simulink model "UZ_EnDat_be4_optimizing_ctrs"  (R2023b)
settings: Solver=FixedStepDiscrete  StartTime=0  StopTime=0.002  RelTol=1e-3
model workspace (MAT data in the model file):
  Select = 0
libraries: hdlsllib x755, simulink x20, simulink_extras x4
(part 1 of 9)
settings Model: DataTypeOverride=Off  SimulationMode=accelerator  NumberOfSteps=10  PacingRate=1000  Creator=ELSYS_PC  LastModifiedBy=ELSYS_PC
settings SolverCC: AlgebraicLoopSolver=TrustRegion
settings DataIOCC: LimitDataPoints=on  SaveOutput=off  SaveTime=off
settings OptimizationCC: BlockReduction=off  ConditionallyExecuteInputs=off  DefaultParameterBehavior=Inlined  InheritOutputTypeSmallerThanSingle=on  LifeSpan=inf
settings DebuggingCC: AlgebraicLoopMsg=error  SingleTaskRateTransMsg=error  UnconnectedInputMsg=warning  UnconnectedOutputMsg=warning  UnconnectedLineMsg=warning  AllowSymbolicDim=off  StrictBusMsg=ErrorOnBusTreatedAsVector  SFUnexpectedBacktrackingDiag=warning  SFNoUnconditionalDefaultTransitionDiag=warning  SFExecutionAtInitializationDiag=none  ArithmeticOperatorsInVariantConditions=warning
settings HardwareCC: ProdBitPerPointer=32  ProdBitPerSizeT=32  ProdBitPerPtrDiffT=32  ProdLargestAtomicFloat=None  ProdIntDivRoundTo=Undefined  ProdEndianess=Unspecified  ProdWordSize=32  ProdHWDeviceType=ASIC/FPGA->ASIC/FPGA  TargetBitPerPointer=64  TargetBitPerSizeT=64  TargetBitPerPtrDiffT=64  TargetLongLongMode=on  TargetIntDivRoundTo=Zero  TargetEndianess=LittleEndian  TargetWordSize=64  TargetHWDeviceType=Custom Processor->MATLAB Host Computer  ProdEqTarget=off
settings ModelReferenceCC: EnableRefExpFcnMdlSchedulingChecks=on
settings SFSimCC: SimUseLocalCustomCode=off  CustomCodeUndefinedFunction=UseInterfaceOnly
settings RTWCC: RTWUseLocalCustomCode=off
settings CodeAppCC: StateflowObjectComments=on
settings GRTTargetCC: TargetLangStandard=C89/C90 (ANSI)  RTWCAPISignals=on  RTWCAPIParams=on
settings ConfigComp: CovScope=ReferencedModels  CovMetricSettings=dw  CovSaveCumulativeToWorkspaceVar=on  CovSaveSingleToWorkspaceVar=on  CovExternalEMLEnable=off  CovSFcnEnable=off  DVTestSuiteOptimization=Auto  DVDetectOutOfBounds=on  DVModelReferenceHarness=on  DVHarnessSource=Signal Editor  DVRebuildModelRepresentation=IfChangeIsDetected

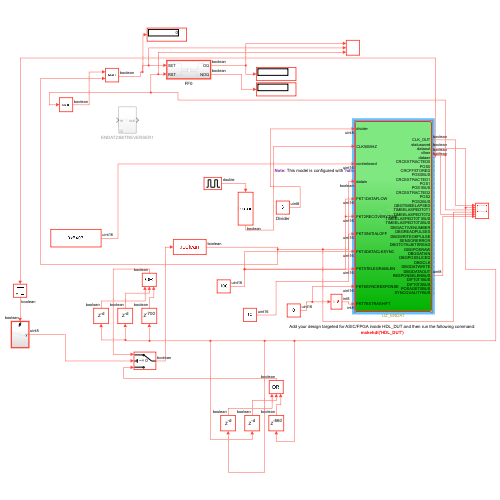
[thumbnail: Simulink's stored preview of the top-level diagram]
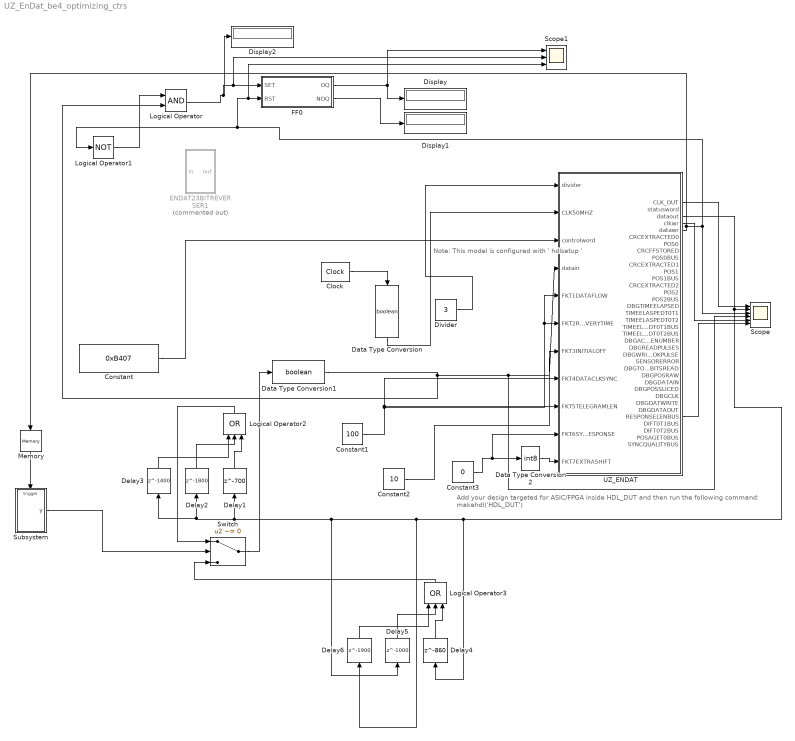
== system UZ_EnDat_be4_optimizing_ctrs ==
  note: Note: This model is configured with ' hdlsetup '
  note: Add your design targeted for ASIC/FPGA inside HDL_DUT and then run the following command:
      | makehdl('HDL_DUT')
  Clock : simulink_extras/Flip Flops/Clock  period=2E-8
  Constant : Constant  Value=0xB407  OutDataTypeStr=uint16  SampleTime=-1
  Constant1 : Constant  Value=100  OutDataTypeStr=uint16  SampleTime=-1
  Constant2 : Constant  Value=10  OutDataTypeStr=uint16  SampleTime=-1
  Constant3 : Constant  Value=0  OutDataTypeStr=uint16  SampleTime=-1
  Data Type Conversion : DataTypeConversion  OutDataTypeStr=boolean  SaturateOnIntegerOverflow=off  RndMeth=Floor
  Data Type Conversion1 : DataTypeConversion  OutDataTypeStr=boolean  SaturateOnIntegerOverflow=off  RndMeth=Floor
  Data Type Conversion2 : DataTypeConversion  OutDataTypeStr=int8  SaturateOnIntegerOverflow=off  RndMeth=Floor
  Delay1 : Delay  DelayLength=700
  Delay2 : Delay  DelayLength=1800
  Delay3 : Delay  DelayLength=1400
  Delay4 : Delay  DelayLength=860
  Delay5 : Delay  DelayLength=1000
  Delay6 : Delay  DelayLength=1900
  Display : Display
  Display1 : Display
  Display2 : Display
  Divider : Constant  Value=3  OutMin=0  OutMax=7  OutDataTypeStr=uint8  SampleTime=-1
  ENDAT23BITREVERSER1 : Subsystem  Commented=on
  FF0 : Subsystem  TreatAsAtomicUnit=on
      settings: LibrarySourceBlock=|
      | hdlsllib/Ports &
      | Subsystems/Triggered
      | Subsystem
  Logical Operator : Logic  AllPortsSameDT=off  OutDataTypeStr=boolean
  Logical Operator1 : Logic  Operator=NOT  AllPortsSameDT=off  OutDataTypeStr=boolean
  Logical Operator2 : Logic  Operator=OR  Inputs=3  AllPortsSameDT=off  OutDataTypeStr=boolean
  Logical Operator3 : Logic  Operator=OR  Inputs=3  AllPortsSameDT=off  OutDataTypeStr=boolean
  Memory : Memory  InheritSampleTime=on
  Scope : Scope  NumInputPorts=6
  Scope1 : Scope  NumInputPorts=3
  Subsystem : Subsystem
  Switch : Switch  Criteria=u2 ~= 0  SaturateOnIntegerOverflow=off  InputSameDT=off
  UZ_ENDAT : Subsystem  TreatAsAtomicUnit=on
  wires:
  Constant/1 -> UZ_ENDAT/3(controlword)
  Data Type Conversion/1 -> UZ_ENDAT/2(CLK50MHZ)
  Divider/1 -> UZ_ENDAT/1(divider)
  Clock/1 -> Data Type Conversion/1
  Data Type Conversion1/1 -> Logical Operator/2, Scope/4, UZ_ENDAT/4(datain)
  Delay1/1 -> Logical Operator2/3
  UZ_ENDAT/1(CLK_OUT) -> Scope/1
  UZ_ENDAT/5(datawr) -> Memory/1, Scope1/3, FF0/2(RST), Logical Operator1/1, Scope/3
  Constant1/1 -> UZ_ENDAT/5(FKT1DATAFLOW), UZ_ENDAT/6(FKT2RECOVERYTIME), UZ_ENDAT/8(FKT4DATACLKSYNC), UZ_ENDAT/9(FKT5TELEGRAMLEN)
  Constant2/1 -> UZ_ENDAT/7(FKT3INITIALOFF)
  FF0/1(OQ) -> Scope1/1, Display/1
  Logical Operator/1 -> Scope1/2, FF0/1(SET), Display2/1
  FF0/2(NOQ) -> Display1/1
  Logical Operator1/1 -> Logical Operator/1
  Delay2/1 -> Logical Operator2/2
  Delay3/1 -> Logical Operator2/1
  Logical Operator2/1 -> Switch/1
  Switch/1 -> Data Type Conversion1/1
  Delay6/1 -> Logical Operator3/1
  Delay5/1 -> Logical Operator3/2
  Logical Operator3/1 -> Switch/3
  Delay4/1 -> Logical Operator3/3
  UZ_ENDAT/3(dataout) -> Delay4/1, Delay6/1, Delay3/1, Delay2/1, Delay1/1, Delay5/1, Scope/2
  Subsystem/1(y) -> Switch/2
  Memory/1 -> Subsystem/Trigger
  UZ_ENDAT/4(clkwr) -> Scope/5
  Constant3/1 -> UZ_ENDAT/10(FKT6SYNCRESPONSE), Data Type Conversion2/1
  Data Type Conversion2/1 -> UZ_ENDAT/11(FKT7EXTRASHIFT)
  UZ_ENDAT/32(RESPONSELENBUS) -> Scope/6

== system UZ_EnDat_be4_optimizing_ctrs/ENDAT23BITREVERSER1 ==
  in : Inport
  16BITREVERSER : Subsystem
  16BITREVERSER1 : Subsystem
  Bit Concat : hdlsllib/Logic and Bit Operations/Bit Concat  numInputs=2
  Bit Shift : hdlsllib/Logic and Bit Operations/Bit Shift  mode=Shift Right Logical  N=8
  Bit Slice : hdlsllib/Logic and Bit Operations/Bit Slice  lidx=15  ridx=0
  Bit Slice1 : hdlsllib/Logic and Bit Operations/Bit Slice  lidx=22  ridx=16
  out : Outport
  wires:
  Bit Concat/1 -> Bit Shift/1
  Bit Shift/1 -> out/1
  in/1 -> Bit Slice1/1, Bit Slice/1
  Bit Slice/1 -> 16BITREVERSER/1(in)
  Bit Slice1/1 -> 16BITREVERSER1/1(in)
  16BITREVERSER/1(out) -> Bit Concat/1
  16BITREVERSER1/1(out) -> Bit Concat/2

== system UZ_EnDat_be4_optimizing_ctrs/FF0 ==
  SET : Inport
  RST : Inport  Port=2
  S-R Flip-Flop : simulink_extras/Flip Flops/S-R Flip-Flop  initial_condition=0
  OQ : Outport
  NOQ : Outport  Port=2
  wires:
  SET/1 -> S-R Flip-Flop/1
  RST/1 -> S-R Flip-Flop/2
  S-R Flip-Flop/1 -> OQ/1
  S-R Flip-Flop/2 -> NOQ/1

== system UZ_EnDat_be4_optimizing_ctrs/Subsystem ==
  Trigger : TriggerPort  VariantControl=(inherit)  PortDimensions=1
  Counter Limited : hdlsllib/Sources/Counter Limited  uplimit=1  tsamp=-1
  y : Outport
  wires:
  Counter Limited/1 -> y/1

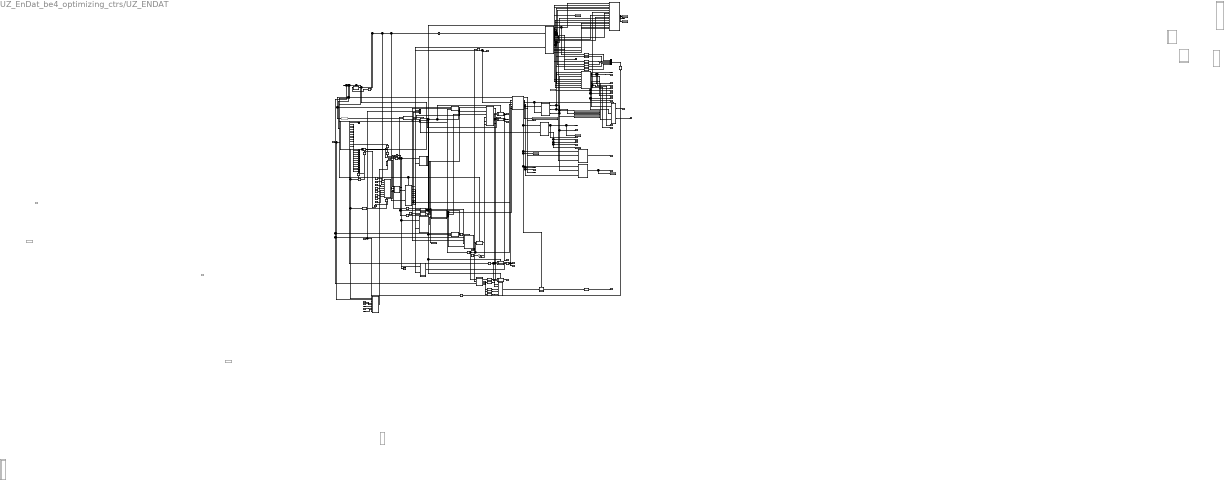
== system UZ_EnDat_be4_optimizing_ctrs/UZ_ENDAT ==
  note: 0=12.5;1=6,25;2=3,125;3=1,5625
  divider : Inport  OutDataTypeStr=uint8  SampleTime=1e-8
  CLK50MHZ : Inport  Port=2  SampleTime=1e-8
  controlword : Inport  Port=3  OutDataTypeStr=uint16  SampleTime=1e-8
  datain : Inport  Port=4  OutDataTypeStr=boolean  SampleTime=1e-8
  FKT1DATAFLOW : Inport  Port=5  OutDataTypeStr=uint16  SampleTime=1e-8
  FKT2RECOVERYTIME : Inport  Port=6  OutDataTypeStr=uint16  SampleTime=1e-8
  FKT3INITIALOFF : Inport  Port=7  OutDataTypeStr=uint16  SampleTime=1e-8
  FKT4DATACLKSYNC : Inport  Port=8  OutDataTypeStr=uint16  SampleTime=1e-8
  FKT5TELEGRAMLEN : Inport  Port=9  OutDataTypeStr=uint16  SampleTime=1e-8
  FKT6SYNCRESPONSE : Inport  Port=10  OutDataTypeStr=uint16  SampleTime=1e-8
  FKT7EXTRASHIFT : Inport  Port=11  OutDataTypeStr=int8  SampleTime=1e-8
  16BIT_SPLITTER1 : Subsystem  Commented=on  TreatAsAtomicUnit=on
  16bitgather : Subsystem
      settings: LibrarySourceBlock=|
      | hdlsllib/Ports &
      | Subsystems/Subsystem
  2CLKDELAY : Delay  DelayLengthSource=Input port  DelayLength=10  DelayLengthUpperLimit=127  PreventDirectFeedthrough=on
      settings: InputPortMap=u0,p1
  3timestorage : Subsystem
      settings: LibrarySourceBlock=|
      | hdlsllib/Ports &
      | Subsystems/Subsystem
  8BIT_SPLITTER : Subsystem  TreatAsAtomicUnit=on
  8BIT_SPLITTER1 : Subsystem  Commented=on  TreatAsAtomicUnit=on
  Bits to Word : hdlsllib/Logic and Bit Operations/Bits to Word
  CLKCNTER_ACT : Subsystem
      settings: LibrarySourceBlock=|
      | hdlsllib/Ports &
      | Subsystems/Subsystem
  CLKCNTER_NOSTOP : Subsystem
      settings: LibrarySourceBlock=|
      | hdlsllib/Ports &
      | Subsystems/Subsystem
  CLKDIV2 : Subsystem  Commented=through
  CLKGEN : Subsystem
  CONTROLWORDRAW : Subsystem
      settings: LibrarySourceBlock=|
      | hdlsllib/Ports &
      | Subsystems/Subsystem
  CONTROLWORDSTORED : Subsystem
      settings: LibrarySourceBlock=|
      | hdlsllib/Ports &
      | Subsystems/Subsystem
  CRC_Check : Subsystem  TreatAsAtomicUnit=on
  Compare To Constant : hdlsllib/Logic and Bit Operations/Compare To Constant  relop===  const=1  OutDataTypeStr=boolean
  Compare To Constant1 : hdlsllib/Logic and Bit Operations/Compare To Constant  relop===  const=1  OutDataTypeStr=boolean
  Compare To Constant2 : hdlsllib/Logic and Bit Operations/Compare To Constant  relop===  const=0  OutDataTypeStr=boolean
  Compare To Constant3 : hdlsllib/Logic and Bit Operations/Compare To Constant  relop=>=  const=3  OutDataTypeStr=boolean
  Constant10 : Constant  Commented=on  Value=3  OutDataTypeStr=fixdt(0,4,0)  SampleTime=-1
  Constant11 : Constant  Commented=on  Value=0xB407  OutDataTypeStr=uint16  SampleTime=-1
  Constant3 : Constant  OutDataTypeStr=boolean  SampleTime=-1
  Constant6 : Constant  Value=51  OutDataTypeStr=uint16  SampleTime=-1
  ControlWordRAM : Constant  Value=0  VectorParams1D=off  OutDataTypeStr=uint8  SampleTime=-1
  DATA2CLOCKSYNCER : Subsystem
  DATA2CLOCKSYNCER1 : Subsystem  Commented=on
  DATAFLOWCHGER : Subsystem
  DIFFBUILDER : Subsystem  TreatAsAtomicUnit=on
  Data Type Conversion : DataTypeConversion  OutDataTypeStr=fixdt(0,4,0)  RndMeth=Nearest
  Data Type Conversion1 : DataTypeConversion  OutDataTypeStr=uint8  SaturateOnIntegerOverflow=off  RndMeth=Floor
  Data Type Conversion{2..12} (11 alike) : DataTypeConversion  OutMax=1  OutDataTypeStr=fixdt(0,1)  SaturateOnIntegerOverflow=off  RndMeth=Floor
  Delay : Delay  DelayLength=10  InitialCondition=0
  Delay1 : Delay  DelayLengthSource=Input port  DelayLengthUpperLimit=127  InitialCondition=0
      settings: InputPortMap=u0,p1
  Delay2 : Delay  DelayLength=1
  Delay3 : Delay  DelayLength=1
  Detect Change : simulink/Logic and Bit Operations/Detect Change  vinit=0  OutDataTypeStr=boolean
      settings: LibrarySourceBlock=|
      | hdlsllib/Logic and Bit
      | Operations/Detect
      | Change
  Display{,1..6,8..11,14..15} (13 alike) : Display
      Display settings: Format=hex (Stored Integer)
      Display1 settings: Format=binary (Stored Integer)
      Display2 settings: Format=binary (Stored Integer)
      Display3 settings: Format=binary (Stored Integer)
      Display4 settings: Format=binary (Stored Integer)
      Display8 settings: Format=hex (Stored Integer)
      Display9 settings: Format=hex (Stored Integer)
  Dual Port RAM System : hdlsllib/HDL RAMs/Dual Port RAM System  RAMType=Dual port  AsyncRead=off  WriteOutputValue=New data  RAMInitialValue=0  allowBusInputs=off  WritesHaveOutput=on  NumReads=0  NumWrites=1  SimulateUsing=Code generation
  EndatControlRAM : Constant  VectorParams1D=off  OutDataTypeStr=uint8  SampleTime=-1
  FKT1 : Constant  Value=2  VectorParams1D=off  OutDataTypeStr=uint8  SampleTime=-1
  FKT2 : Constant  Value=3  VectorParams1D=off  OutDataTypeStr=uint8  SampleTime=-1
  FKT3 : Constant  Commented=on  Value=4  VectorParams1D=off  OutDataTypeStr=uint8  SampleTime=-1
  FKT4 : Constant  Value=5  VectorParams1D=off  OutDataTypeStr=uint8  SampleTime=-1
  FKT5 : Constant  Value=6  VectorParams1D=off  OutDataTypeStr=uint8  SampleTime=-1
  FKT6 : Constant  Value=7  VectorParams1D=off  OutDataTypeStr=uint8  SampleTime=-1
  FKT7 : Constant  Value=8  VectorParams1D=off  OutDataTypeStr=uint8  SampleTime=-1
  INITIALOFF : Subsystem
  Logical Operator : Logic  AllPortsSameDT=off  OutDataTypeStr=boolean
  Logical Operator1 : Logic  AllPortsSameDT=off  OutDataTypeStr=boolean
  Logical Operator10 : Logic  Operator=NOT  Inputs=3  AllPortsSameDT=off  OutDataTypeStr=boolean
  Logical Operator{2..4,27} (4 alike) : Logic  Operator=NOT  AllPortsSameDT=off  OutDataTypeStr=boolean
  Logical Operator25 : Logic  Commented=through  Operator=NOT  AllPortsSameDT=off  OutDataTypeStr=boolean
  Logical Operator6 : Logic  Operator=NOT  Inputs=3  AllPortsSameDT=off  OutDataTypeStr=boolean
  Logical Operator8 : Logic  Inputs=3  AllPortsSameDT=off  OutDataTypeStr=boolean
  ManualSerialize : Subsystem
      settings: LibrarySourceBlock=|
      | hdlsllib/Ports &
      | Subsystems/Subsystem
  ManualSerialize1 : Subsystem  Commented=on
      settings: LibrarySourceBlock=|
      | hdlsllib/Ports &
      | Subsystems/Subsystem
  Memory : Memory  InheritSampleTime=on
  OUTPUTCONTROLCONTINIOUS : Subsystem
      settings: LibrarySourceBlock=|
      | hdlsllib/Ports &
      | Subsystems/Subsystem
  RAM_SELECTOR : MultiPortSwitch  DataPortOrder=Zero-based contiguous  Inputs=8  zeroidx=on  OutDataTypeStr=uint8  SaturateOnIntegerOverflow=off  InputSameDT=off
  RAM_SELECTOR1 : MultiPortSwitch  DataPortOrder=Zero-based contiguous  Inputs=8  zeroidx=on  SaturateOnIntegerOverflow=off  InputSameDT=off
  RAM_SELECTOR2 : MultiPortSwitch  Commented=on  DataPortOrder=Zero-based contiguous  Inputs=16  DataPortForDefault=Additional data port  zeroidx=on  SaturateOnIntegerOverflow=off  InputSameDT=off
  RECOVERYTIMESELECTOR : Subsystem
  RESPONSESLICER3X : Subsystem
  Scope2 : Scope  NumInputPorts=2
  SetZero32modified : Subsystem  Commented=on
  SetZeroBool : Subsystem
  SetZeroBool1 : Subsystem
  SetZeroBool2 : Subsystem
  SetZeroBool3 : Subsystem
  SetZeroBool4 : Subsystem
  SetZeroBool5 : Subsystem
  Signal Specification : SignalSpecification  OutDataTypeStr=uint16
  Storage16 : Subsystem
      settings: LibrarySourceBlock=|
      | hdlsllib/Ports &
      | Subsystems/Subsystem
  Subsystem1 : Subsystem
  Subsystem2 : Subsystem
  Subsystem6 : Subsystem
  Terminator{,1,4,12..17,19..25} (16 alike) : Terminator
  Vector Concatenate : Concatenate  NumInputs=6
  Vector Concatenate1 : Concatenate  NumInputs=5
  ageprovider : Subsystem
      settings: LibrarySourceBlock=|
      | hdlsllib/Ports &
      | Subsystems/Subsystem
  ramselektor : Subsystem  TreatAsAtomicUnit=on
      settings: LibrarySourceBlock=|
      | hdlsllib/Ports &
      | Subsystems/Triggered
      | Subsystem
  responseslicer5 : Subsystem  Commented=on  TreatAsAtomicUnit=on
      settings: LibrarySourceBlock=|
      | hdlsllib/Ports &
      | Subsystems/Subsystem
  signalquality : Subsystem
      settings: LibrarySourceBlock=|
      | hdlsllib/Ports &
      | Subsystems/Subsystem
  timingprovider : Subsystem
      settings: LibrarySourceBlock=|
      | hdlsllib/Ports &
      | Subsystems/Subsystem
  CLK_OUT : Outport  VectorParamsAs1DForOutWhenUnconnected=off
  statusword : Outport  Port=2  OutDataTypeStr=uint16  VectorParamsAs1DForOutWhenUnconnected=off
  dataout : Outport  Port=3  OutDataTypeStr=boolean  VectorParamsAs1DForOutWhenUnconnected=off
  clkwr : Outport  Port=4  OutDataTypeStr=boolean  VectorParamsAs1DForOutWhenUnconnected=off
  datawr : Outport  Port=5  OutDataTypeStr=boolean  VectorParamsAs1DForOutWhenUnconnected=off
  CRCEXTRACTED0 : Outport  Port=6  OutDataTypeStr=uint8  VectorParamsAs1DForOutWhenUnconnected=off
  POS0 : Outport  Port=7  OutDataTypeStr=uint32  VectorParamsAs1DForOutWhenUnconnected=off
  CRCFFSTORED : Outport  Port=8  OutDataTypeStr=uint8  VectorParamsAs1DForOutWhenUnconnected=off
  POS0BUS : Outport  Port=9  OutDataTypeStr=uint32  VectorParamsAs1DForOutWhenUnconnected=off
  CRCEXTRACTED1 : Outport  Port=10  OutDataTypeStr=uint8  VectorParamsAs1DForOutWhenUnconnected=off
  POS1 : Outport  Port=11  OutDataTypeStr=uint32  VectorParamsAs1DForOutWhenUnconnected=off
  POS1BUS : Outport  Port=12  OutDataTypeStr=uint32  VectorParamsAs1DForOutWhenUnconnected=off
  CRCEXTRACTED2 : Outport  Port=13  OutDataTypeStr=uint8  VectorParamsAs1DForOutWhenUnconnected=off
  POS2 : Outport  Port=14  OutDataTypeStr=uint32  VectorParamsAs1DForOutWhenUnconnected=off
  POS2BUS : Outport  Port=15  OutDataTypeStr=uint32  VectorParamsAs1DForOutWhenUnconnected=off
  DBGTIMEELAPSED : Outport  Port=16  VectorParamsAs1DForOutWhenUnconnected=off
  TIMEELASPEDT0T1 : Outport  Port=17  VectorParamsAs1DForOutWhenUnconnected=off
  TIMEELASPEDT0T2 : Outport  Port=18  VectorParamsAs1DForOutWhenUnconnected=off
  TIMEELASPEDT0T1BUS : Outport  Port=19  VectorParamsAs1DForOutWhenUnconnected=off
  TIMEELASPEDT0T2BUS : Outport  Port=20  VectorParamsAs1DForOutWhenUnconnected=off
  DBGACTIVENUMBER : Outport  Port=21  OutDataTypeStr=uint8  VectorParamsAs1DForOutWhenUnconnected=off
  DBGREADPULSES : Outport  Port=22  OutDataTypeStr=boolean  VectorParamsAs1DForOutWhenUnconnected=off
  DBGWRITEOKPULSE : Outport  Port=23  OutDataTypeStr=boolean  VectorParamsAs1DForOutWhenUnconnected=off
  SENSORERROR : Outport  Port=24  OutDataTypeStr=boolean  VectorParamsAs1DForOutWhenUnconnected=off
  DBGTOTALBITSREAD : Outport  Port=25  VectorParamsAs1DForOutWhenUnconnected=off
  DBGPOSRAW : Outport  Port=26  OutDataTypeStr=uint64  VectorParamsAs1DForOutWhenUnconnected=off
  DBGDATAIN : Outport  Port=27  OutDataTypeStr=boolean  VectorParamsAs1DForOutWhenUnconnected=off
  DBGPOSSLICED : Outport  Port=28  OutDataTypeStr=uint32  VectorParamsAs1DForOutWhenUnconnected=off
  DBGCLK : Outport  Port=29  VectorParamsAs1DForOutWhenUnconnected=off
  DBGDATWRITE : Outport  Port=30  VectorParamsAs1DForOutWhenUnconnected=off
  DBGDATAOUT : Outport  Port=31  OutDataTypeStr=boolean  VectorParamsAs1DForOutWhenUnconnected=off
  RESPONSELENBUS : Outport  Port=32  VectorParamsAs1DForOutWhenUnconnected=off
  DIFT0T1BUS : Outport  Port=33  OutDataTypeStr=int32  VectorParamsAs1DForOutWhenUnconnected=off
  DIFT0T2BUS : Outport  Port=34  OutDataTypeStr=int32  VectorParamsAs1DForOutWhenUnconnected=off
  POSAGET0BUS : Outport  Port=35  VectorParamsAs1DForOutWhenUnconnected=off
  SYNCQUALITYBUS : Outport  Port=36  VectorParamsAs1DForOutWhenUnconnected=off
  wires:
  CONTROLWORDSTORED/1(DATAOUT0) -> 16bitgather/1(in1), Data Type Conversion4/1
  timingprovider/1(timeelapsed2cycl) -> Display14/1, TIMEELASPEDT0T2/1, TIMEELASPEDT0T2BUS/1
  timingprovider/2(timeelapsed1cycl) -> TIMEELASPEDT0T1BUS/1, Display11/1, TIMEELASPEDT0T1/1, DBGTIMEELAPSED/1
  Storage16/1(out) -> Display/1, Subsystem2/3(DATA)
  Data Type Conversion/1 -> RECOVERYTIMESELECTOR/1(In1), DATA2CLOCKSYNCER/1(In1), DATAFLOWCHGER/1(CLKSEL), CLKGEN/1(CLKSEL)
  CONTROLWORDSTORED/6(DATAOUT5) -> Data Type Conversion9/1
  CONTROLWORDSTORED/4(DATAOUT3) -> 16bitgather/4(DATAOUT4), Data Type Conversion7/1
  CONTROLWORDSTORED/14(DATAOUT13) -> Terminator/1
  8BIT_SPLITTER/9(DATAOUT8) -> Terminator4/1
  SetZeroBool1/1(valueout) -> INITIALOFF/4(DATA)
  Memory/1 -> ramselektor/1(In1)
  ageprovider/1(posage) -> POSAGET0BUS/1
  RESPONSESLICER3X/2(payload) -> POS0BUS/1, POS0/1, DBGPOSSLICED/1, DIFFBUILDER/1(DATAT0)
  CONTROLWORDRAW/5(DATAOUT4) -> Terminator16/1
  Data Type Conversion8/1 -> Vector Concatenate/5
  DATAFLOWCHGER/1(Output) -> OUTPUTCONTROLCONTINIOUS/2(CLKS2DATAFLOWCHG)
  CONTROLWORDSTORED/5(DATAOUT4) -> 16bitgather/5(DATAOUT5), Data Type Conversion8/1
  Logical Operator27/1 -> SetZeroBool4/2(setzero), SetZeroBool3/2(setzero), SetZeroBool5/2(setzero), SetZeroBool2/2(setzero)
  CONTROLWORDRAW/7(DATAOUT6) -> Terminator23/1
  Vector Concatenate/1 -> Bits to Word/1
  Constant6/1 -> Subsystem6/1(In1)
  SetZeroBool4/1(valueout) -> DBGDATWRITE/1, datawr/1
  ManualSerialize/3(wrok) -> Subsystem1/Enable, signalquality/1(wrok), Display6/1, ageprovider/1(wrok), timingprovider/1(wrok), DIFFBUILDER/Trigger, 3timestorage/2(wrok)
  Data Type Conversion7/1 -> Vector Concatenate/4
  CLKCNTER_ACT/1(CNT) -> OUTPUTCONTROLCONTINIOUS/1(CLKCNT), Compare To Constant3/1
  Detect Change/1 -> Logical Operator/1
  Data Type Conversion9/1 -> Vector Concatenate/6
  RESPONSESLICER3X/5(CRC2) -> CRCEXTRACTED2/1
  Data Type Conversion6/1 -> Vector Concatenate/3
  DIFFBUILDER/2(DIFT2T0) -> DIFT0T2BUS/1
  CONTROLWORDRAW/6(DATAOUT5) -> Terminator22/1
  Data Type Conversion4/1 -> Vector Concatenate/1
  8BIT_SPLITTER/6(DATAOUT5) -> Subsystem6/2(FACTOR)
  OUTPUTCONTROLCONTINIOUS/1(CLKOFF) -> Subsystem2/4(reset), ManualSerialize/5(clkoff), SetZeroBool/2(setzero)
  8BIT_SPLITTER/4(DATAOUT3) -> RECOVERYTIMESELECTOR/2(FAKTOR)
  Delay2/1 -> Logical Operator8/1
  8BIT_SPLITTER/3(DATAOUT2) -> DATAFLOWCHGER/2(FACTOR)
  RESPONSESLICER3X/1(CRC) -> CRCEXTRACTED0/1
  CONTROLWORDRAW/1(DATAOUT0) -> Terminator12/1
  CLK50MHZ/1 -> CRC_Check/3(clk), Subsystem2/1(CLK), CLKCNTER_ACT/1(CLK), CLKCNTER_NOSTOP/1(CLK), CLKDIV2/1(CLK1), ManualSerialize/1(CLK), SetZeroBool1/Trigger, 8BIT_SPLITTER/Trigger, ramselektor/Trigger, timingprovider/2(clk), CONTROLWORDRAW/1(CLK)
  CONTROLWORDRAW/9(DATAOUT8) -> Terminator25/1
  Subsystem6/1(Out1) -> OUTPUTCONTROLCONTINIOUS/3(CLK2ENDOFTRANSMISSION)
  3timestorage/1(t0) -> signalquality/2(payload), DBGPOSRAW/1, Display1/1, RESPONSESLICER3X/1(DATA)
  FKT4/1 -> RAM_SELECTOR/6
  INITIALOFF/4(CLKWR_OUT) -> SetZeroBool2/1(valin)
  FKT5/1 -> RAM_SELECTOR/7
  DIFFBUILDER/1(DIFT1T0) -> DIFT0T1BUS/1
  SetZeroBool/1(valueout) -> SetZeroBool5/Trigger, SetZeroBool2/Trigger, CLKCNTER_ACT/2(CLK2CNT), INITIALOFF/2(CLK), SetZeroBool4/Trigger, SetZeroBool3/Trigger
  CONTROLWORDSTORED/11(DATAOUT10) -> RESPONSESLICER3X/7(25BIT), 16bitgather/11(In11)
  CLKGEN/1(RESCLK) -> Subsystem2/2(SLOWCLCK), SetZeroBool/1(valin), SetZeroBool/Trigger, CLKCNTER_NOSTOP/2(CLK2CNT)
  INITIALOFF/3(DATA_OUT) -> SetZeroBool3/1(valin)
  Data Type Conversion5/1 -> Vector Concatenate/2
  FKT2/1 -> RAM_SELECTOR/5
  CONTROLWORDRAW/13(DATAOUT12) -> Logical Operator27/1
  INITIALOFF/2(DATAWR_OUT) -> SetZeroBool4/1(valin)
  Logical Operator/1 -> Dual Port RAM System/3
  FKT6SYNCRESPONSE/1 -> RAM_SELECTOR1/8
  FKT5TELEGRAMLEN/1 -> RAM_SELECTOR1/7
  CONTROLWORDRAW/4(DATAOUT3) -> Terminator15/1
  CONTROLWORDRAW/2(DATAOUT1) -> Terminator13/1
  INITIALOFF/1(CLK_OUT) -> SetZeroBool5/1(valin)
  Data Type Conversion12/1 -> Vector Concatenate1/5
  CONTROLWORDRAW/15(DATAOUT14) -> Terminator17/1
  FKT2RECOVERYTIME/1 -> RAM_SELECTOR1/5
  Constant3/1 -> Logical Operator25/1
  Logical Operator25/1 -> INITIALOFF/5(CLKWR)
  Data Type Conversion2/1 -> Vector Concatenate1/1
  Delay/1 -> RAM_SELECTOR1/3
  CRC_Check/6(CRC5) -> Data Type Conversion12/1
  EndatControlRAM/1 -> RAM_SELECTOR/3
  CRC_Check/3(CRC2) -> Data Type Conversion3/1
  CONTROLWORDRAW/11(DATAOUT10) -> Terminator20/1
  CONTROLWORDRAW/12(DATAOUT11) -> Terminator19/1
  SetZeroBool5/1(valueout) -> 2CLKDELAY/1
  Storage16/2(wrok) -> 16bitgather/14(wrok), Logical Operator6/1
  RESPONSESLICER3X/4(payload1) -> POS1/1, DIFFBUILDER/2(DATAT1), POS1BUS/1
  RESPONSESLICER3X/6(payload2) -> POS2BUS/1, POS2/1, DIFFBUILDER/3(DATAT2)
  CRC_Check/2(CRC1) -> Data Type Conversion2/1
  ManualSerialize/2(valueout) -> 3timestorage/1(DATA), Display4/1
  ManualSerialize/4(dbg2) -> signalquality/3(dbg2), DBGTOTALBITSREAD/1, RESPONSELENBUS/1
  Data Type Conversion3/1 -> Vector Concatenate1/2
  Subsystem1/1(out) -> Data Type Conversion1/1
  FKT6/1 -> RAM_SELECTOR/8
  DATA2CLOCKSYNCER/1(Out1) -> 2CLKDELAY/2
  Data Type Conversion11/1 -> Vector Concatenate1/4
  SetZeroBool2/1(valueout) -> clkwr/1
  FKT3INITIALOFF/1 -> INITIALOFF/6(FACTOR)
  CONTROLWORDRAW/16(DATAOUT15) -> Logical Operator3/1
  Logical Operator4/1 -> ManualSerialize/4(recieving), SetZeroBool1/2(setzero), CRC_Check/1(set)
  8BIT_SPLITTER/5(DATAOUT4) -> DATA2CLOCKSYNCER/2(FAKTOR)
  8BIT_SPLITTER/2(DATAOUT1) -> Storage16/1(Data)
  CONTROLWORDRAW/8(DATAOUT7) -> Terminator24/1
  Subsystem2/1(valin) -> SetZeroBool1/1(valin)
  CONTROLWORDRAW/10(DATAOUT9) -> Terminator21/1
  ManualSerialize/5(dbg1) -> DBGWRITEOKPULSE/1
  CRC_Check/5(CRC4) -> Data Type Conversion11/1
  CONTROLWORDRAW/3(DATAOUT2) -> Terminator14/1
  Data Type Conversion1/1 -> CRCFFSTORED/1
  3timestorage/2(t-1) -> Display2/1, RESPONSESLICER3X/2(DATA1)
  FKT1/1 -> RAM_SELECTOR/4
  Data Type Conversion10/1 -> Vector Concatenate1/3
  divider/1 -> Data Type Conversion/1
  Dual Port RAM System/1 -> Terminator1/1
  FKT7/1 -> RAM_SELECTOR/9
  RESPONSESLICER3X/3(CRC1) -> CRCEXTRACTED1/1
  ManualSerialize/1(dbg) -> DBGREADPULSES/1
  CRC_Check/4(CRC3) -> Data Type Conversion10/1
  Dual Port RAM System/2 -> 8BIT_SPLITTER/1(DATAIN)
  FKT1DATAFLOW/1 -> RAM_SELECTOR1/4
  FKT4DATACLKSYNC/1 -> RAM_SELECTOR1/6
  ControlWordRAM/1 -> RAM_SELECTOR/2
  RECOVERYTIMESELECTOR/1(Out1) -> OUTPUTCONTROLCONTINIOUS/6(RECOVERYTIME)
  CONTROLWORDSTORED/2(DATAOUT1) -> 16bitgather/2(DATAOUT1), Data Type Conversion5/1
  Bits to Word/1 -> Delay/1
  CONTROLWORDSTORED/3(DATAOUT2) -> 16bitgather/3(DATAOUT3), Data Type Conversion6/1
  OUTPUTCONTROLCONTINIOUS/2(DATAINV) -> INITIALOFF/3(DATAWR), Logical Operator4/1
  RESPONSESLICER3X/7(sensorerror) -> 16bitgather/6(DATAOUT6), SENSORERROR/1
  RAM_SELECTOR/1 -> Dual Port RAM System/2, Dual Port RAM System/4
  signalquality/1(amoundofsyncs) -> SYNCQUALITYBUS/1, Display5/1
  RESPONSESLICER3X/8(DBGACTIVENUMBER) -> Display10/1, DBGACTIVENUMBER/1
  CONTROLWORDSTORED/9(DATAOUT8) -> 16bitgather/9(DATAOUT9), RESPONSESLICER3X/5(21BIT)
  SetZeroBool3/1(valueout) -> dataout/1, DBGDATAOUT/1
  controlword/1 -> RAM_SELECTOR1/2, CONTROLWORDRAW/2(DATA)
  FKT7EXTRASHIFT/1 -> Scope2/1, RAM_SELECTOR1/9
  Delay1/1 -> ManualSerialize/3(DATA), DBGDATAIN/1
  OUTPUTCONTROLCONTINIOUS/3(RESETCNT) -> CLKCNTER_NOSTOP/3(ResetCNT), CLKCNTER_ACT/3(ResetCNT)
  CONTROLWORDSTORED/7(DATAOUT6) -> 16bitgather/7(DATAOUT7), ageprovider/3(altmode), Display15/1
  CONTROLWORDSTORED/8(DATAOUT7) -> 16bitgather/8(DATAOUT8), RESPONSESLICER3X/4(19BIT)
  8BIT_SPLITTER/8(DATAOUT7) -> ManualSerialize/6(FKT7EXTRASHIFTER), Scope2/2
  16bitgather/1(statusword) -> Display8/1, statusword/1, Display9/1
  2CLKDELAY/1 -> DBGCLK/1, CLK_OUT/1, ManualSerialize/2(SLOWCLCK)
  ManualSerialize/6(beginrecieving) -> ageprovider/2(recieving)
  Logical Operator8/1 -> Storage16/2(Write), Logical Operator10/1
  CONTROLWORDSTORED/12(DATAOUT11) -> 16bitgather/12(DATAOUT11), RESPONSESLICER3X/8(27BIT)
  CONTROLWORDSTORED/10(DATAOUT9) -> 16bitgather/10(DATAOUT10), RESPONSESLICER3X/6(23BIT)
  ramselektor/1(SEL) -> RAM_SELECTOR1/1, Detect Change/1, Compare To Constant/1, Compare To Constant1/1, Memory/1, Compare To Constant2/1, 8BIT_SPLITTER/2(SEL), RAM_SELECTOR/1
  3timestorage/3(t-2) -> Display3/1, RESPONSESLICER3X/3(DATA2)
  datain/1 -> Delay1/1, CRC_Check/2(data)
  Logical Operator10/1 -> OUTPUTCONTROLCONTINIOUS/4(OPENCOM)
  CLKDIV2/1(CLK/2) -> CLKGEN/2(CLK1)
  CONTROLWORDRAW/14(DATAOUT13) -> Delay2/1
  CONTROLWORDSTORED/13(DATAOUT12) -> 16bitgather/13(DATAOUT12)
  Compare To Constant2/1 -> CONTROLWORDSTORED/1(CLK)
  8BIT_SPLITTER/1(DATAOUT0) -> CONTROLWORDSTORED/2(DATA)
  Vector Concatenate1/1 -> Subsystem1/1(in)
  Compare To Constant1/1 -> Delay3/1
  8BIT_SPLITTER/7(DATAOUT6) -> Delay1/2
  CLKGEN/2(SLOWCLK) -> INITIALOFF/1(CLKAUX)
  CONTROLWORDSTORED/16(DATAOUT15) -> 16bitgather/16(DATAOUT15)
  CONTROLWORDSTORED/15(DATAOUT14) -> 16bitgather/15(DATAOUT14)
  Logical Operator3/1 -> Logical Operator1/1
  Logical Operator1/1 -> Logical Operator2/1
  Compare To Constant/1 -> Logical Operator1/2
  Logical Operator2/1 -> Logical Operator/2
  Delay3/1 -> Logical Operator8/2
  Signal Specification/1 -> Dual Port RAM System/1
  RAM_SELECTOR1/1 -> Signal Specification/1
  Compare To Constant3/1 -> Subsystem2/Enable
  Logical Operator6/1 -> Logical Operator8/3
  CLKCNTER_NOSTOP/1(CNT) -> OUTPUTCONTROLCONTINIOUS/5(CLKCNTNOSTOP)

== system UZ_EnDat_be4_optimizing_ctrs/ENDAT23BITREVERSER1/16BITREVERSER ==
  in : Inport
  Bit Concat : hdlsllib/Logic and Bit Operations/Bit Concat  numInputs=4
  Bit Slice : hdlsllib/Logic and Bit Operations/Bit Slice  lidx=3  ridx=0
  Bit Slice1 : hdlsllib/Logic and Bit Operations/Bit Slice  lidx=7  ridx=4
  Bit Slice2 : hdlsllib/Logic and Bit Operations/Bit Slice  lidx=11  ridx=8
  Bit Slice3 : hdlsllib/Logic and Bit Operations/Bit Slice  lidx=15  ridx=12
  out : Outport
  wires:
  in/1 -> Bit Slice/1, Bit Slice3/1, Bit Slice2/1, Bit Slice1/1
  Bit Slice1/1 -> Bit Concat/2
  Bit Slice/1 -> Bit Concat/1
  Bit Slice2/1 -> Bit Concat/3
  Bit Slice3/1 -> Bit Concat/4
  Bit Concat/1 -> out/1

== system UZ_EnDat_be4_optimizing_ctrs/ENDAT23BITREVERSER1/16BITREVERSER1 ==
  in : Inport
  Bit Concat : hdlsllib/Logic and Bit Operations/Bit Concat  numInputs=4
  Bit Slice : hdlsllib/Logic and Bit Operations/Bit Slice  lidx=3  ridx=0
  Bit Slice1 : hdlsllib/Logic and Bit Operations/Bit Slice  lidx=7  ridx=4
  Bit Slice2 : hdlsllib/Logic and Bit Operations/Bit Slice  lidx=11  ridx=8
  Bit Slice3 : hdlsllib/Logic and Bit Operations/Bit Slice  lidx=15  ridx=12
  out : Outport
  wires:
  in/1 -> Bit Slice/1, Bit Slice3/1, Bit Slice2/1, Bit Slice1/1
  Bit Slice1/1 -> Bit Concat/2
  Bit Slice/1 -> Bit Concat/1
  Bit Slice2/1 -> Bit Concat/3
  Bit Slice3/1 -> Bit Concat/4
  Bit Concat/1 -> out/1

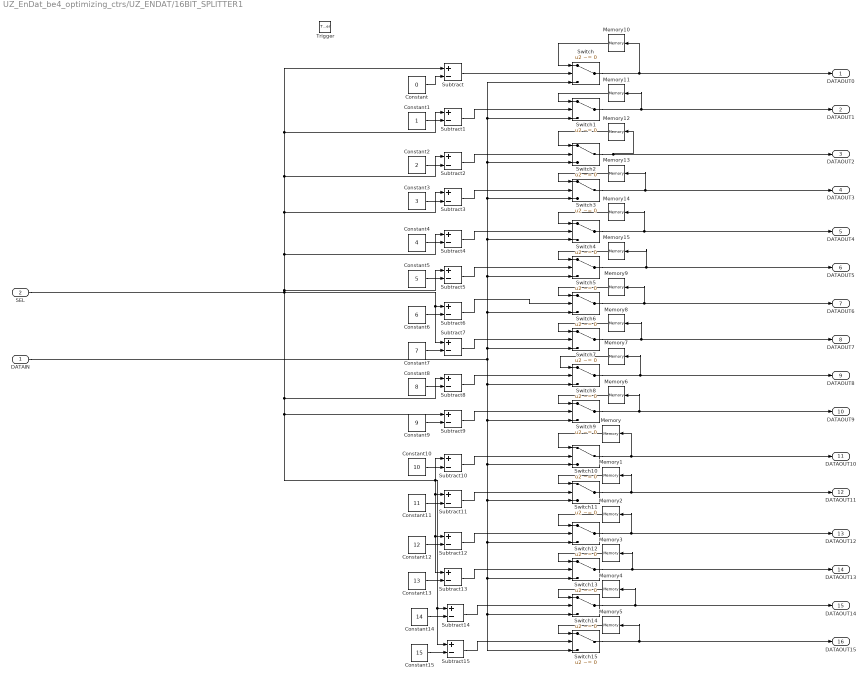
== system UZ_EnDat_be4_optimizing_ctrs/UZ_ENDAT/16BIT_SPLITTER1 ==
  DATAIN : Inport
  SEL : Inport  Port=2  OutDataTypeStr=fixdt(0,4,0)
  Trigger : TriggerPort  TriggerType=falling  VariantControl=(inherit)  OutputDataType=int8  InitialTriggerSignalState=positive
  Constant : Constant  Value=0  OutDataTypeStr=fixdt(0,4,0)  SampleTime=-1
  Constant1 : Constant  OutDataTypeStr=fixdt(0,4,0)  SampleTime=-1
  Constant10 : Constant  Value=10  OutDataTypeStr=fixdt(0,4,0)  SampleTime=-1
  Constant11 : Constant  Value=11  OutDataTypeStr=fixdt(0,4,0)  SampleTime=-1
  Constant12 : Constant  Value=12  OutDataTypeStr=fixdt(0,4,0)  SampleTime=-1
  Constant13 : Constant  Value=13  OutDataTypeStr=fixdt(0,4,0)  SampleTime=-1
  Constant14 : Constant  Value=14  OutDataTypeStr=fixdt(0,4,0)  SampleTime=-1
  Constant15 : Constant  Value=15  OutDataTypeStr=fixdt(0,4,0)  SampleTime=-1
  Constant2 : Constant  Value=2  OutDataTypeStr=fixdt(0,4,0)  SampleTime=-1
  Constant3 : Constant  Value=3  OutDataTypeStr=fixdt(0,4,0)  SampleTime=-1
  Constant4 : Constant  Value=4  OutDataTypeStr=fixdt(0,4,0)  SampleTime=-1
  Constant5 : Constant  Value=5  OutDataTypeStr=fixdt(0,4,0)  SampleTime=-1
  Constant6 : Constant  Value=6  OutDataTypeStr=fixdt(0,4,0)  SampleTime=-1
  Constant7 : Constant  Value=7  OutDataTypeStr=fixdt(0,4,0)  SampleTime=-1
  Constant8 : Constant  Value=8  OutDataTypeStr=fixdt(0,4,0)  SampleTime=-1
  Constant9 : Constant  Value=9  OutDataTypeStr=fixdt(0,4,0)  SampleTime=-1
  Memory{,1..8,10..11} (11 alike) : Memory  InheritSampleTime=on
  Memory{9,12..15} (5 alike) : Memory  InitialCondition=100  InheritSampleTime=on  LinearizeAsDelay=on
  Subtract{,1..9,11..15} (15 alike) : Sum  Inputs=+-  OutDataTypeStr=fixdt(0,4,0)
  Subtract10 : Sum  Inputs=+-  AccumDataTypeStr=fixdt(0,4,0)
  Switch{,1..15} (16 alike) : Switch  Criteria=u2 ~= 0  SaturateOnIntegerOverflow=off  InputSameDT=off
  DATAOUT0 : Outport  InitialOutput=0
  DATAOUT1 : Outport  Port=2  InitialOutput=0
  DATAOUT2 : Outport  Port=3  InitialOutput=0
  DATAOUT3 : Outport  Port=4  InitialOutput=0
  DATAOUT4 : Outport  Port=5  InitialOutput=0
  DATAOUT5 : Outport  Port=6  InitialOutput=0
  DATAOUT6 : Outport  Port=7  InitialOutput=0
  DATAOUT7 : Outport  Port=8  InitialOutput=0
  DATAOUT8 : Outport  Port=9  InitialOutput=0
  DATAOUT9 : Outport  Port=10  InitialOutput=0
  DATAOUT10 : Outport  Port=11  InitialOutput=0
  DATAOUT11 : Outport  Port=12  InitialOutput=0
  DATAOUT12 : Outport  Port=13  InitialOutput=0
  DATAOUT13 : Outport  Port=14  InitialOutput=0
  DATAOUT14 : Outport  Port=15  InitialOutput=0
  DATAOUT15 : Outport  Port=16  InitialOutput=0
  wires:
  Switch/1 -> Memory10/1, DATAOUT0/1
  Switch1/1 -> Memory11/1, DATAOUT1/1
  Switch3/1 -> Memory13/1, DATAOUT3/1
  Switch2/1 -> Memory12/1, DATAOUT2/1
  Switch5/1 -> Memory15/1, DATAOUT5/1
  Switch4/1 -> Memory14/1, DATAOUT4/1
  Switch7/1 -> Memory8/1, DATAOUT7/1
  Switch6/1 -> Memory9/1, DATAOUT6/1
  Switch9/1 -> Memory6/1, DATAOUT9/1
  Switch10/1 -> Memory/1, DATAOUT10/1
  Switch11/1 -> Memory1/1, DATAOUT11/1
  Switch8/1 -> Memory7/1, DATAOUT8/1
  Switch12/1 -> Memory2/1, DATAOUT12/1
  Switch15/1 -> Memory5/1, DATAOUT15/1
  Switch13/1 -> Memory3/1, DATAOUT13/1
  Switch14/1 -> Memory4/1, DATAOUT14/1
  Constant/1 -> Subtract/2
  Subtract/1 -> Switch/2
  Subtract1/1 -> Switch1/2
  Constant1/1 -> Subtract1/2
  Constant2/1 -> Subtract2/2
  Subtract2/1 -> Switch2/2
  Constant3/1 -> Subtract3/2
  Subtract3/1 -> Switch3/2
  Constant4/1 -> Subtract4/2
  Subtract4/1 -> Switch4/2
  Constant5/1 -> Subtract5/2
  Subtract5/1 -> Switch5/2
  Constant6/1 -> Subtract6/2
  Subtract6/1 -> Switch6/2
  Constant7/1 -> Subtract7/2
  Subtract7/1 -> Switch7/2
  Constant8/1 -> Subtract8/2
  Subtract8/1 -> Switch8/2
  Constant9/1 -> Subtract9/2
  Subtract9/1 -> Switch9/2
  Constant10/1 -> Subtract10/2
  Subtract10/1 -> Switch10/2
  Constant11/1 -> Subtract11/2
  Subtract11/1 -> Switch11/2
  Constant12/1 -> Subtract12/2
  Subtract12/1 -> Switch12/2
  Constant13/1 -> Subtract13/2
  Subtract13/1 -> Switch13/2
  Constant14/1 -> Subtract14/2
  Subtract14/1 -> Switch14/2
  Constant15/1 -> Subtract15/2
  SEL/1 -> Subtract15/1, Subtract14/1, Subtract13/1, Subtract12/1, Subtract11/1, Subtract10/1, Subtract9/1, Subtract8/1, Subtract7/1, Subtract6/1, Subtract5/1, Subtract4/1, Subtract3/1, Subtract2/1, Subtract1/1, Subtract/1
  Subtract15/1 -> Switch15/2
  DATAIN/1 -> Switch4/3, Switch3/3, Switch2/3, Switch1/3, Switch/3, Switch5/3, Switch6/3, Switch7/3, Switch9/3, Switch10/3, Switch11/3, Switch12/3, Switch14/3, Switch15/3, Switch13/3, Switch8/3
  Memory/1 -> Switch10/1
  Memory1/1 -> Switch11/1
  Memory2/1 -> Switch12/1
  Memory3/1 -> Switch13/1
  Memory4/1 -> Switch14/1
  Memory5/1 -> Switch15/1
  Memory6/1 -> Switch9/1
  Memory7/1 -> Switch8/1
  Memory8/1 -> Switch7/1
  Memory9/1 -> Switch6/1
  Memory10/1 -> Switch/1
  Memory11/1 -> Switch1/1
  Memory12/1 -> Switch2/1
  Memory13/1 -> Switch3/1
  Memory14/1 -> Switch4/1
  Memory15/1 -> Switch5/1

== system UZ_EnDat_be4_optimizing_ctrs/UZ_ENDAT/16bitgather ==
  in1 : Inport
  DATAOUT1 : Inport  Port=2
  DATAOUT3 : Inport  Port=3
  DATAOUT4 : Inport  Port=4
  DATAOUT5 : Inport  Port=5
  DATAOUT6 : Inport  Port=6
  DATAOUT7 : Inport  Port=7
  DATAOUT8 : Inport  Port=8
  DATAOUT9 : Inport  Port=9
  DATAOUT10 : Inport  Port=10
  In11 : Inport  Port=11
  DATAOUT11 : Inport  Port=12
  DATAOUT12 : Inport  Port=13
  wrok : Inport  Port=14
  DATAOUT14 : Inport  Port=15
  DATAOUT15 : Inport  Port=16
  Bits to Word1 : hdlsllib/Logic and Bit Operations/Bits to Word
  Data Type Conversion{1..16} (16 alike) : DataTypeConversion  OutMax=1  OutDataTypeStr=fixdt(0,1)  SaturateOnIntegerOverflow=off  RndMeth=Floor
  Vector Concatenate1 : Concatenate  NumInputs=16
  statusword : Outport
  wires:
  in1/1 -> Data Type Conversion1/1
  DATAOUT1/1 -> Data Type Conversion2/1
  DATAOUT3/1 -> Data Type Conversion3/1
  DATAOUT4/1 -> Data Type Conversion10/1
  DATAOUT5/1 -> Data Type Conversion11/1
  DATAOUT6/1 -> Data Type Conversion12/1
  DATAOUT7/1 -> Data Type Conversion4/1
  DATAOUT8/1 -> Data Type Conversion5/1
  DATAOUT9/1 -> Data Type Conversion6/1
  DATAOUT10/1 -> Data Type Conversion7/1
  In11/1 -> Data Type Conversion8/1
  DATAOUT11/1 -> Data Type Conversion9/1
  DATAOUT12/1 -> Data Type Conversion13/1
  wrok/1 -> Data Type Conversion14/1
  DATAOUT14/1 -> Data Type Conversion15/1
  Bits to Word1/1 -> statusword/1
  Vector Concatenate1/1 -> Bits to Word1/1
  Data Type Conversion11/1 -> Vector Concatenate1/5
  Data Type Conversion3/1 -> Vector Concatenate1/3
  Data Type Conversion2/1 -> Vector Concatenate1/2
  Data Type Conversion1/1 -> Vector Concatenate1/1
  Data Type Conversion12/1 -> Vector Concatenate1/6
  Data Type Conversion10/1 -> Vector Concatenate1/4
  Data Type Conversion4/1 -> Vector Concatenate1/7
  DATAOUT15/1 -> Data Type Conversion16/1
  Data Type Conversion5/1 -> Vector Concatenate1/8
  Data Type Conversion6/1 -> Vector Concatenate1/9
  Data Type Conversion7/1 -> Vector Concatenate1/10
  Data Type Conversion8/1 -> Vector Concatenate1/11
  Data Type Conversion9/1 -> Vector Concatenate1/12
  Data Type Conversion13/1 -> Vector Concatenate1/13
  Data Type Conversion14/1 -> Vector Concatenate1/14
  Data Type Conversion15/1 -> Vector Concatenate1/15
  Data Type Conversion16/1 -> Vector Concatenate1/16

== system UZ_EnDat_be4_optimizing_ctrs/UZ_ENDAT/3timestorage ==
  DATA : Inport
  wrok : Inport  Port=2  OutMin=0  OutMax=1  OutDataTypeStr=boolean
  Compare To Constant : hdlsllib/Logic and Bit Operations/Compare To Constant  relop===  const=0  OutDataTypeStr=boolean
  Compare To Constant1 : hdlsllib/Logic and Bit Operations/Compare To Constant  relop===  const=1  OutDataTypeStr=boolean
  Compare To Constant2 : hdlsllib/Logic and Bit Operations/Compare To Constant  relop===  const=2  OutDataTypeStr=boolean
  Detect Increase2 : simulink/Logic and Bit Operations/Detect Increase  vinit=0.0  OutDataTypeStr=boolean
      settings: LibrarySourceBlock=|
      | hdlsllib/Logic and Bit
      | Operations/Detect
      | Increase
  Detect Increase3 : simulink/Logic and Bit Operations/Detect Increase  vinit=0.0  OutDataTypeStr=boolean
      settings: LibrarySourceBlock=|
      | hdlsllib/Logic and Bit
      | Operations/Detect
      | Increase
  Detect Increase4 : simulink/Logic and Bit Operations/Detect Increase  vinit=0.0  OutDataTypeStr=boolean
      settings: LibrarySourceBlock=|
      | hdlsllib/Logic and Bit
      | Operations/Detect
      | Increase
  Multiport Switch : MultiPortSwitch  DataPortOrder=Zero-based contiguous  zeroidx=on  RndMeth=Simplest  SaturateOnIntegerOverflow=off  InputSameDT=off
  Multiport Switch1 : MultiPortSwitch  DataPortOrder=Zero-based contiguous  zeroidx=on  RndMeth=Simplest  SaturateOnIntegerOverflow=off  InputSameDT=off
  Multiport Switch2 : MultiPortSwitch  DataPortOrder=Zero-based contiguous  zeroidx=on  RndMeth=Simplest  SaturateOnIntegerOverflow=off  InputSameDT=off
  Storage1 : Subsystem
      settings: LibrarySourceBlock=|
      | hdlsllib/Ports &
      | Subsystems/Subsystem
  Storage2 : Subsystem
      settings: LibrarySourceBlock=|
      | hdlsllib/Ports &
      | Subsystems/Subsystem
  Storage20 : Subsystem
      settings: LibrarySourceBlock=|
      | hdlsllib/Ports &
      | Subsystems/Subsystem
  Triggered Subsystem : Subsystem  TreatAsAtomicUnit=on
      settings: LibrarySourceBlock=|
      | hdlsllib/Ports &
      | Subsystems/Triggered
      | Subsystem
  t0 : Outport
  t-1 : Outport  Port=2
  t-2 : Outport  Port=3
  wires:
  Triggered Subsystem/1(Out1) -> Multiport Switch2/1, Multiport Switch1/1, Multiport Switch/1, Compare To Constant/1, Compare To Constant1/1, Compare To Constant2/1
  wrok/1 -> Triggered Subsystem/Trigger
  DATA/1 -> Storage2/1(Data), Storage1/1(Data), Storage20/1(Data)
  Compare To Constant/1 -> Detect Increase4/1
  Compare To Constant1/1 -> Detect Increase3/1
  Compare To Constant2/1 -> Detect Increase2/1
  Storage20/1(out) -> Multiport Switch2/4, Multiport Switch1/3, Multiport Switch/2
  Storage1/1(out) -> Multiport Switch2/2, Multiport Switch1/4, Multiport Switch/3
  Multiport Switch/1 -> t0/1
  Storage2/1(out) -> Multiport Switch/4, Multiport Switch1/2, Multiport Switch2/3
  Multiport Switch1/1 -> t-1/1
  Multiport Switch2/1 -> t-2/1
  Detect Increase2/1 -> Storage2/2(Write)
  Detect Increase3/1 -> Storage1/2(Write)
  Detect Increase4/1 -> Storage20/2(Write)

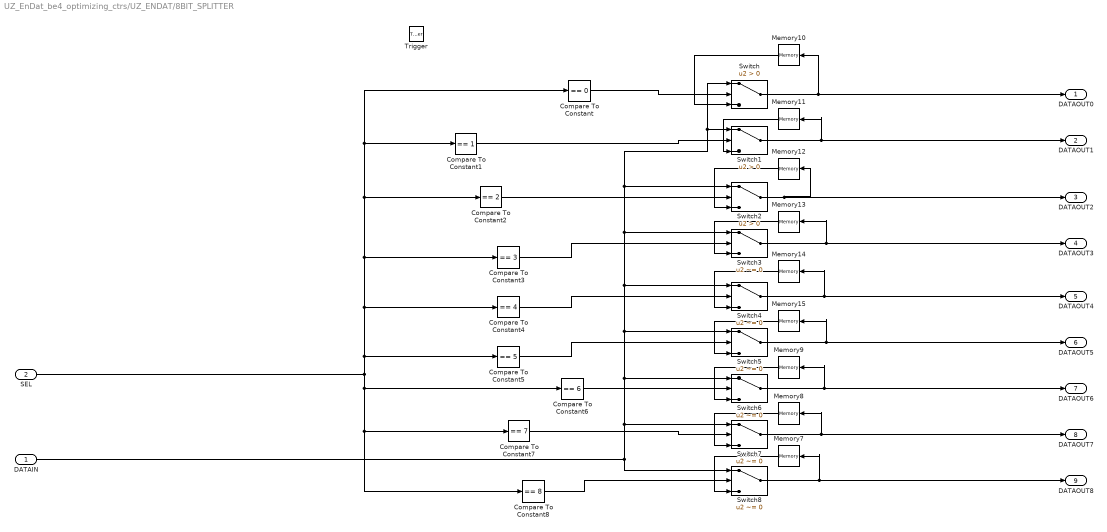
== system UZ_EnDat_be4_optimizing_ctrs/UZ_ENDAT/8BIT_SPLITTER ==
  DATAIN : Inport
  SEL : Inport  Port=2  OutDataTypeStr=fixdt(0,4,0)
  Trigger : TriggerPort  TriggerType=falling  VariantControl=(inherit)  OutputDataType=int8  InitialTriggerSignalState=positive
  Compare To Constant : hdlsllib/Logic and Bit Operations/Compare To Constant  relop===  const=0  OutDataTypeStr=boolean
  Compare To Constant1 : hdlsllib/Logic and Bit Operations/Compare To Constant  relop===  const=1  OutDataTypeStr=boolean
  Compare To Constant2 : hdlsllib/Logic and Bit Operations/Compare To Constant  relop===  const=2  OutDataTypeStr=boolean
  Compare To Constant3 : hdlsllib/Logic and Bit Operations/Compare To Constant  relop===  const=3  OutDataTypeStr=boolean
  Compare To Constant4 : hdlsllib/Logic and Bit Operations/Compare To Constant  relop===  const=4  OutDataTypeStr=boolean
  Compare To Constant5 : hdlsllib/Logic and Bit Operations/Compare To Constant  relop===  const=5  OutDataTypeStr=boolean
  Compare To Constant6 : hdlsllib/Logic and Bit Operations/Compare To Constant  relop===  const=6  OutDataTypeStr=boolean
  Compare To Constant7 : hdlsllib/Logic and Bit Operations/Compare To Constant  relop===  const=7  OutDataTypeStr=boolean
  Compare To Constant8 : hdlsllib/Logic and Bit Operations/Compare To Constant  relop===  const=8  OutDataTypeStr=boolean
  Memory{7..8,10..11} (4 alike) : Memory  InheritSampleTime=on
  Memory{9,12..15} (5 alike) : Memory  InitialCondition=100  InheritSampleTime=on  LinearizeAsDelay=on
  Switch : Switch  Criteria=u2 > Threshold  SaturateOnIntegerOverflow=off  InputSameDT=off
  Switch1 : Switch  Criteria=u2 > Threshold  SaturateOnIntegerOverflow=off  InputSameDT=off
  Switch2 : Switch  Criteria=u2 > Threshold  SaturateOnIntegerOverflow=off  InputSameDT=off
  Switch{3..8} (6 alike) : Switch  Criteria=u2 ~= 0  SaturateOnIntegerOverflow=off  InputSameDT=off
  DATAOUT0 : Outport  InitialOutput=0
  DATAOUT1 : Outport  Port=2  InitialOutput=0
  DATAOUT2 : Outport  Port=3  InitialOutput=0
  DATAOUT3 : Outport  Port=4  InitialOutput=0
  DATAOUT4 : Outport  Port=5  InitialOutput=0
  DATAOUT5 : Outport  Port=6  InitialOutput=0
  DATAOUT6 : Outport  Port=7  InitialOutput=0
  DATAOUT7 : Outport  Port=8  InitialOutput=0
  DATAOUT8 : Outport  Port=9  InitialOutput=0
  wires:
  Switch/1 -> Memory10/1, DATAOUT0/1
  Switch1/1 -> Memory11/1, DATAOUT1/1
  Switch3/1 -> Memory13/1, DATAOUT3/1
  Switch2/1 -> Memory12/1, DATAOUT2/1
  Switch5/1 -> Memory15/1, DATAOUT5/1
  Switch4/1 -> Memory14/1, DATAOUT4/1
  Switch7/1 -> Memory8/1, DATAOUT7/1
  Switch6/1 -> Memory9/1, DATAOUT6/1
  Switch8/1 -> Memory7/1, DATAOUT8/1
  Compare To Constant7/1 -> Switch7/2
  ? -> ?
  SEL/1 -> Compare To Constant6/1, Compare To Constant8/1, Compare To Constant7/1, Compare To Constant5/1, Compare To Constant4/1, Compare To Constant2/1, Compare To Constant1/1, Compare To Constant/1, Compare To Constant3/1
  DATAIN/1 -> Switch8/1, Switch7/1, Switch6/1, Switch5/1, Switch4/1, Switch3/1, Switch2/1, Switch1/1, Switch/1
  Memory7/1 -> Switch8/3
  Memory8/1 -> Switch7/3
  Memory9/1 -> Switch6/3
  Memory10/1 -> Switch/3
  Memory11/1 -> Switch1/3
  Memory12/1 -> Switch2/3
  Memory13/1 -> Switch3/3
  Memory14/1 -> Switch4/3
  Memory15/1 -> Switch5/3
  Compare To Constant/1 -> Switch/2
  Compare To Constant1/1 -> Switch1/2
  Compare To Constant2/1 -> Switch2/2
  Compare To Constant3/1 -> Switch3/2
  Compare To Constant4/1 -> Switch4/2
  Compare To Constant5/1 -> Switch5/2
  Compare To Constant6/1 -> Switch6/2
  Compare To Constant8/1 -> Switch8/2

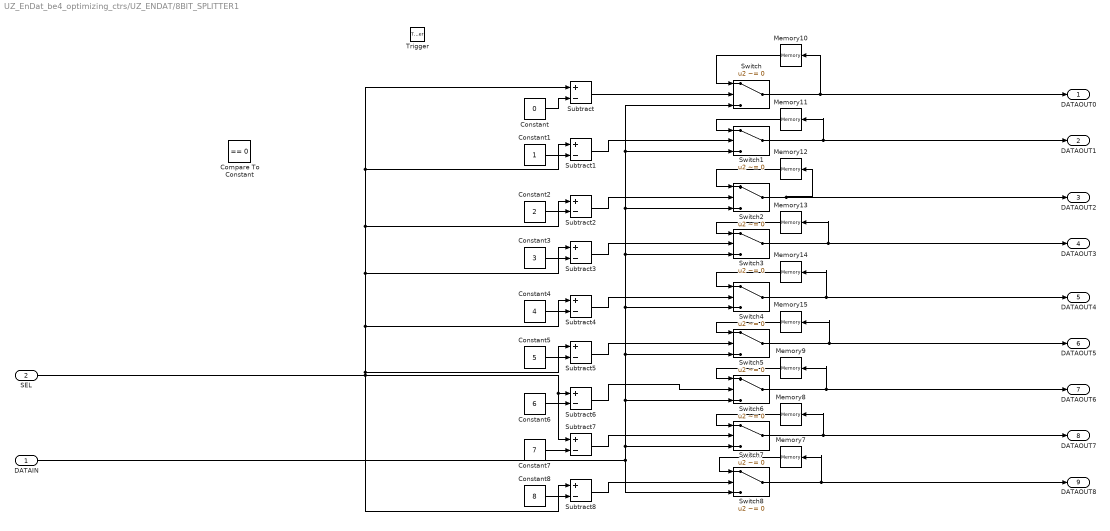
== system UZ_EnDat_be4_optimizing_ctrs/UZ_ENDAT/8BIT_SPLITTER1 ==
  DATAIN : Inport
  SEL : Inport  Port=2  OutDataTypeStr=fixdt(0,4,0)
  Trigger : TriggerPort  TriggerType=falling  VariantControl=(inherit)  OutputDataType=int8  InitialTriggerSignalState=positive
  Compare To Constant : hdlsllib/Logic and Bit Operations/Compare To Constant  relop===  const=0  OutDataTypeStr=boolean
  Constant : Constant  Value=0  OutDataTypeStr=fixdt(0,4,0)  SampleTime=-1
  Constant1 : Constant  OutDataTypeStr=fixdt(0,4,0)  SampleTime=-1
  Constant2 : Constant  Value=2  OutDataTypeStr=fixdt(0,4,0)  SampleTime=-1
  Constant3 : Constant  Value=3  OutDataTypeStr=fixdt(0,4,0)  SampleTime=-1
  Constant4 : Constant  Value=4  OutDataTypeStr=fixdt(0,4,0)  SampleTime=-1
  Constant5 : Constant  Value=5  OutDataTypeStr=fixdt(0,4,0)  SampleTime=-1
  Constant6 : Constant  Value=6  OutDataTypeStr=fixdt(0,4,0)  SampleTime=-1
  Constant7 : Constant  Value=7  OutDataTypeStr=fixdt(0,4,0)  SampleTime=-1
  Constant8 : Constant  Value=8  OutDataTypeStr=fixdt(0,4,0)  SampleTime=-1
  Memory{7..8,10..11} (4 alike) : Memory  InheritSampleTime=on
  Memory{9,12..15} (5 alike) : Memory  InitialCondition=100  InheritSampleTime=on  LinearizeAsDelay=on
  Subtract{,1..8} (9 alike) : Sum  Inputs=+-  OutDataTypeStr=fixdt(0,4,0)
  Switch{,1..8} (9 alike) : Switch  Criteria=u2 ~= 0  SaturateOnIntegerOverflow=off  InputSameDT=off
  DATAOUT0 : Outport  InitialOutput=0
  DATAOUT1 : Outport  Port=2  InitialOutput=0
  DATAOUT2 : Outport  Port=3  InitialOutput=0
  DATAOUT3 : Outport  Port=4  InitialOutput=0
  DATAOUT4 : Outport  Port=5  InitialOutput=0
  DATAOUT5 : Outport  Port=6  InitialOutput=0
  DATAOUT6 : Outport  Port=7  InitialOutput=0
  DATAOUT7 : Outport  Port=8  InitialOutput=0
  DATAOUT8 : Outport  Port=9  InitialOutput=0
  wires:
  Switch/1 -> Memory10/1, DATAOUT0/1
  Switch1/1 -> Memory11/1, DATAOUT1/1
  Switch3/1 -> Memory13/1, DATAOUT3/1
  Switch2/1 -> Memory12/1, DATAOUT2/1
  Switch5/1 -> Memory15/1, DATAOUT5/1
  Switch4/1 -> Memory14/1, DATAOUT4/1
  Switch7/1 -> Memory8/1, DATAOUT7/1
  Switch6/1 -> Memory9/1, DATAOUT6/1
  Switch8/1 -> Memory7/1, DATAOUT8/1
  Constant/1 -> Subtract/2
  Subtract/1 -> Switch/2
  Subtract1/1 -> Switch1/2
  Constant1/1 -> Subtract1/2
  Constant2/1 -> Subtract2/2
  Subtract2/1 -> Switch2/2
  Constant3/1 -> Subtract3/2
  Subtract3/1 -> Switch3/2
  Constant4/1 -> Subtract4/2
  Subtract4/1 -> Switch4/2
  Constant5/1 -> Subtract5/2
  Subtract5/1 -> Switch5/2
  Constant6/1 -> Subtract6/2
  Subtract6/1 -> Switch6/2
  Constant7/1 -> Subtract7/2
  Subtract7/1 -> Switch7/2
  Constant8/1 -> Subtract8/2
  Subtract8/1 -> Switch8/2
  ? -> ?
  SEL/1 -> Subtract8/1, Subtract7/1, Subtract6/1, Subtract5/1, Subtract4/1, Subtract3/1, Subtract2/1, Subtract1/1, Subtract/1
  DATAIN/1 -> Switch4/3, Switch3/3, Switch2/3, Switch1/3, Switch/3, Switch5/3, Switch6/3, Switch7/3, Switch8/3
  Memory7/1 -> Switch8/1
  Memory8/1 -> Switch7/1
  Memory9/1 -> Switch6/1
  Memory10/1 -> Switch/1
  Memory11/1 -> Switch1/1
  Memory12/1 -> Switch2/1
  Memory13/1 -> Switch3/1
  Memory14/1 -> Switch4/1
  Memory15/1 -> Switch5/1

== system UZ_EnDat_be4_optimizing_ctrs/UZ_ENDAT/CLKCNTER_ACT ==
  CLK : Inport
  CLK2CNT : Inport  Port=2
  ResetCNT : Inport  Port=3  OutDataTypeStr=boolean
  Delay1 : Delay  DelayLength=1
  Positional_Counter : Subsystem  TreatAsAtomicUnit=on
      settings: LibrarySourceBlock=|
      | hdlsllib/Ports &
      | Subsystems/Triggered
      | Subsystem
  SetZero32modified : Subsystem
  CNT : Outport
  wires:
  CLK2CNT/1 -> Positional_Counter/Trigger
  Delay1/1 -> Positional_Counter/1(valueout), CNT/1
  SetZero32modified/1(valueout) -> Delay1/1
  CLK/1 -> SetZero32modified/Trigger
  Positional_Counter/1(divider) -> SetZero32modified/1(valin)
  ResetCNT/1 -> SetZero32modified/2(setzero)

== system UZ_EnDat_be4_optimizing_ctrs/UZ_ENDAT/CLKCNTER_NOSTOP ==
  CLK : Inport
  CLK2CNT : Inport  Port=2
  ResetCNT : Inport  Port=3  OutDataTypeStr=boolean
  Delay1 : Delay  DelayLength=1
  Positional_Counter : Subsystem  TreatAsAtomicUnit=on
      settings: LibrarySourceBlock=|
      | hdlsllib/Ports &
      | Subsystems/Triggered
      | Subsystem
  SetZero32modified : Subsystem
  CNT : Outport
  wires:
  Delay1/1 -> SetZero32modified/1(valin), CNT/1
  CLK2CNT/1 -> Positional_Counter/Trigger
  ResetCNT/1 -> SetZero32modified/2(setzero)
  Positional_Counter/1(divider) -> Delay1/1
  CLK/1 -> SetZero32modified/Trigger
  SetZero32modified/1(valueout) -> Positional_Counter/1(valueout)

== system UZ_EnDat_be4_optimizing_ctrs/UZ_ENDAT/CLKDIV2 ==
  CLK1 : Inport  OutDataTypeStr=boolean
  Delay : Delay  DelayLength=1
  Logical Operator1 : Logic  Operator=NOT  AllPortsSameDT=off  OutDataTypeStr=boolean
  Triggered Subsystem : Subsystem  TreatAsAtomicUnit=on
      settings: LibrarySourceBlock=|
      | hdlsllib/Ports &
      | Subsystems/Triggered
      | Subsystem
  CLK/2 : Outport  OutDataTypeStr=boolean  VectorParamsAs1DForOutWhenUnconnected=off
  wires:
  Logical Operator1/1 -> CLK/2/1, Delay/1
  CLK1/1 -> Triggered Subsystem/Trigger
  Triggered Subsystem/1(OUT) -> Logical Operator1/1
  Delay/1 -> Triggered Subsystem/1(IN)

== system UZ_EnDat_be4_optimizing_ctrs/UZ_ENDAT/CLKGEN ==
  CLKSEL : Inport
  CLK1 : Inport  Port=2
  CLKDIV1 : Subsystem
  CLKDIV3 : Subsystem
  CLKDIV4 : Subsystem
  CLKDIV5 : Subsystem
  CLKDIV6 : Subsystem
  CLKDIV7 : Subsystem
  CLKDIV8 : Subsystem
  CLKDIV9 : Subsystem
  Multiport Switch : MultiPortSwitch  DataPortOrder=Zero-based contiguous  Inputs=7  DataPortIndices={8,16,32,64}  zeroidx=on  SaturateOnIntegerOverflow=off  InputSameDT=off
  RESCLK : Outport
  SLOWCLK : Outport  Port=2
  wires:
  CLKDIV8/1(CLK/2) -> CLKDIV9/1(CLK1), Multiport Switch/7
  Multiport Switch/1 -> RESCLK/1
  CLKDIV4/1(CLK/2) -> CLKDIV5/1(CLK1), Multiport Switch/3
  CLKDIV5/1(CLK/2) -> CLKDIV6/1(CLK1), Multiport Switch/4
  CLKDIV9/1(CLK/2) -> Multiport Switch/8, SLOWCLK/1
  CLKDIV1/1(CLK/2) -> CLKDIV3/1(CLK1)
  CLKDIV7/1(CLK/2) -> CLKDIV8/1(CLK1), Multiport Switch/6
  CLKDIV3/1(CLK/2) -> CLKDIV4/1(CLK1), Multiport Switch/2
  CLKDIV6/1(CLK/2) -> CLKDIV7/1(CLK1), Multiport Switch/5
  CLK1/1 -> CLKDIV1/1(CLK1)
  CLKSEL/1 -> Multiport Switch/1
